simulink model "prob_7"  (R2020b)
settings: Solver=VariableStepAuto  StartTime=0.0  StopTime=10.0  RelTol=1e-3
settings Model: Creator=Akshay A H  LastModifiedBy=Akshay A H

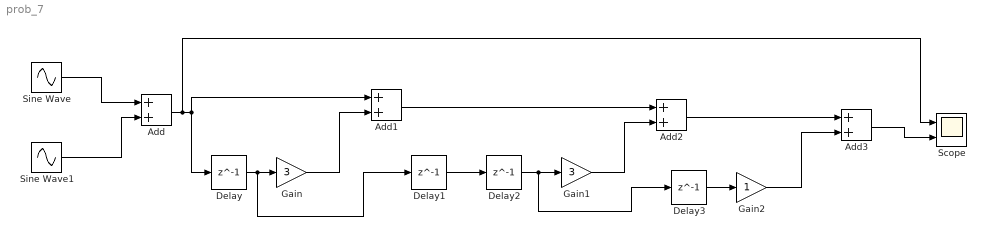
== system prob_7 ==
  Add{,1..3} (4 alike) : Sum
  Delay{,1..3} (4 alike) : Delay  DelayLength=1
  Gain : Gain  Gain=3
  Gain1 : Gain  Gain=3
  Gain2 : Gain
  Scope : Scope  NumInputPorts=2
  Sine Wave : Sin  SampleTime=0
  Sine Wave1 : Sin  Amplitude=0.00001  Frequency=2000  SampleTime=0
  wires:
  Sine Wave/1 -> Add/1
  Sine Wave1/1 -> Add/2
  Add/1 -> Scope/1, Delay/1, Add1/1
  Delay/1 -> Delay1/1, Gain/1
  Gain/1 -> Add1/2
  Delay1/1 -> Delay2/1
  Delay2/1 -> Delay3/1, Gain1/1
  Add1/1 -> Add2/1
  Gain1/1 -> Add2/2
  Add2/1 -> Add3/1
  Delay3/1 -> Gain2/1
  Gain2/1 -> Add3/2
  Add3/1 -> Scope/2
